simulink model "plantaNeural"  (Simulink 7.4)
settings: Solver=ode45  StartTime=0.0  StopTime=10000  RelTol=1e-3
undefined symbols (not defined in the file or in its folder): now
libraries: neural x29, simulink_extras x2
settings Model: Creator=marco  LastModifiedBy=marco

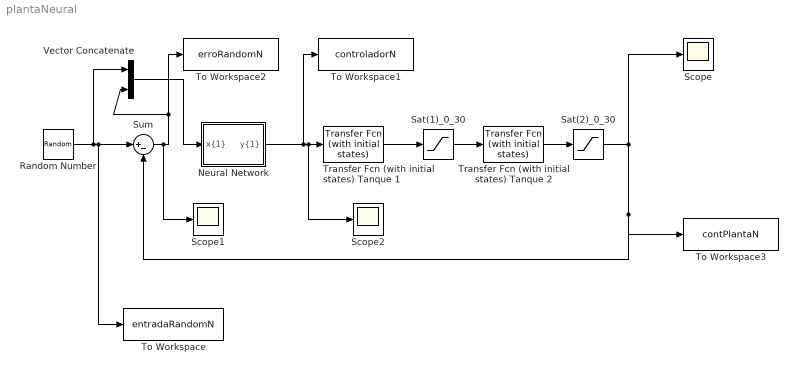
== system plantaNeural ==
  Neural Network : Subsystem
  Random Number : RandomNumber  Mean=15  Variance=15  Seed=round(now)  SampleTime=500
  Sat(1)_0_30 : Saturate  UpperLimit=30  LowerLimit=0  SampleTime=0.1  OutDataType=fixdt(1, 16)  OutScaling=2^0
  Sat(2)_0_30 : Saturate  UpperLimit=30  LowerLimit=0  SampleTime=0.1  OutDataType=fixdt(1, 16)  OutScaling=2^0
  Scope : Scope
  Scope1 : Scope
  Scope2 : Scope
      settings: YMin=4  YMax=5.5  SaveName=ScopeData2
  Sum : Sum  Inputs=|+-  OutDataType=fixdt(1, 16)  OutScaling=2^0  SampleTime=0.1
  To Workspace : ToWorkspace  VariableName=entradaRandomN  SampleTime=0.1  SaveFormat=Array
  To Workspace1 : ToWorkspace  VariableName=controladorN  SampleTime=0.1  SaveFormat=Array
  To Workspace2 : ToWorkspace  VariableName=erroRandomN  SampleTime=0.1  SaveFormat=Array
  To Workspace3 : ToWorkspace  VariableName=contPlantaN  SampleTime=0.1  SaveFormat=Array
  Transfer Fcn (with initial states) Tanque 1 : simulink_extras/Additional Linear/Transfer Fcn (with initial states)  SystemSampleTime=-1  N=[0.2964]  D="[1  0.0656]"  X0=0
  Transfer Fcn (with initial states) Tanque 2 : simulink_extras/Additional Linear/Transfer Fcn (with initial states)  SystemSampleTime=-1  N=[0.0656]  D="[1  0.0656]"  X0=0
  Vector Concatenate : Concatenate  Mode=Vector
  wires:
  Transfer Fcn (with initial states) Tanque 1/1 -> Sat(1)_0_30/1
  Sum/1 -> Scope1/1, To Workspace2/1, Vector Concatenate/2
  Transfer Fcn (with initial states) Tanque 2/1 -> Sat(2)_0_30/1
  Neural Network/1("y{1}") -> To Workspace1/1, Transfer Fcn (with initial states) Tanque 1/1, Scope2/1
  Random Number/1 -> To Workspace/1, Sum/1, Vector Concatenate/1
  Sat(1)_0_30/1 -> Transfer Fcn (with initial states) Tanque 2/1
  Sat(2)_0_30/1 -> Scope/1, Sum/2, To Workspace3/1
  Vector Concatenate/1 -> Neural Network/1("x{1}")

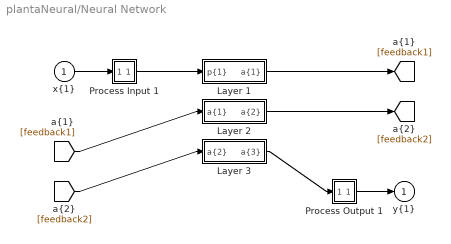
== system plantaNeural/Neural Network ==
  "x{1}" : Inport  PortDimensions=2  SampleTime=1
  Layer 1 : Subsystem
  Layer 2 : Subsystem
  Layer 3 : Subsystem
  Process Input 1 : Subsystem
  Process Output 1 : Subsystem
  "y{1}" : Outport  InitialOutput=0
  wires:
  "x{1}"/1 -> Process Input 1/1(x)
  Process Output 1/1(y) -> "y{1}"/1
  Process Input 1/1(p) -> Layer 1/1("p{1}")
  Layer 1/1("a{1}") -> [feedback1]
  [feedback1] -> Layer 2/1("a{1} ")
  Layer 2/1("a{2}") -> [feedback2]
  [feedback2] -> Layer 3/1("a{2} ")
  Layer 3/1("a{3}") -> Process Output 1/1(a)

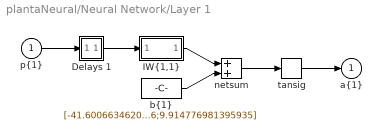
== system plantaNeural/Neural Network/Layer 1 ==
  "p{1}" : Inport  PortDimensions=2  SampleTime=1
  Delays 1 : Subsystem
      mask Display: disp('TDL')
  "IW{1,1}" : Subsystem
      mask Display: disp('weight')
  "b{1}" : Constant  Value=[-41.600663462015341;-13.867070844846031;-1.0368982298681877;-25.663752606811631;65.028796099680704;3.5608850337005888;6.4712500253222389;61.743011559162341;7.1136119483346736;9.914776981395935]
      mask Display: disp('bias')
  netsum : Sum  Inputs=2  OutDataType=sfix(16)  OutScaling=2^0  SaturateOnIntegerOverflow=on  InputSameDT=on  OutDataTypeStr=Inherit: Same as first input
  tansig : neural/Transfer Functions/tansig  SystemSampleTime=-1
  "a{1}" : Outport  InitialOutput=[0;0;0;0;0;0;0;0;0;0]
  wires:
  "p{1}"/1 -> Delays 1/1("p{1}")
  Delays 1/1("pd{1,1}") -> "IW{1,1}"/1("pd{1,1}")
  "IW{1,1}"/1("iz{1,1}") -> netsum/1
  "b{1}"/1 -> netsum/2
  netsum/1 -> tansig/1
  tansig/1 -> "a{1}"/1

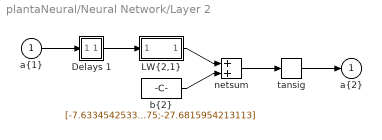
== system plantaNeural/Neural Network/Layer 2 ==
  "a{1} " : Inport  PortDimensions=10  SampleTime=1
  Delays 1 : Subsystem
      mask Display: disp('TDL')
  "LW{2,1}" : Subsystem
      mask Display: disp('weight')
  "b{2}" : Constant  Value=[-7.6334542533188312;-15.605769004106929;9.5386103916769969;-0.097339973816270103;36.782799143926788;8.2018066341292926;15.153030458866333;4.2679298498601739;36.406304506237475;-27.6815954213113]
      mask Display: disp('bias')
  netsum : Sum  Inputs=2  OutDataType=sfix(16)  OutScaling=2^0  SaturateOnIntegerOverflow=on  InputSameDT=on  OutDataTypeStr=Inherit: Same as first input
  tansig : neural/Transfer Functions/tansig  SystemSampleTime=-1
  "a{2}" : Outport  InitialOutput=[0;0;0;0;0;0;0;0;0;0]
  wires:
  "a{1} "/1 -> Delays 1/1("p{2}")
  Delays 1/1("pd{2,1}") -> "LW{2,1}"/1("ad{2,1}")
  "LW{2,1}"/1("lz{2,1}") -> netsum/1
  "b{2}"/1 -> netsum/2
  netsum/1 -> tansig/1
  tansig/1 -> "a{2}"/1

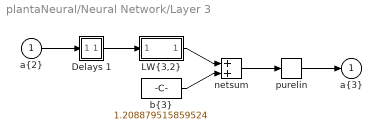
== system plantaNeural/Neural Network/Layer 3 ==
  "a{2} " : Inport  PortDimensions=10  SampleTime=1
  Delays 1 : Subsystem
      mask Display: disp('TDL')
  "LW{3,2}" : Subsystem
      mask Display: disp('weight')
  "b{3}" : Constant  Value=1.208879515859524
      mask Display: disp('bias')
  netsum : Sum  Inputs=2  OutDataType=sfix(16)  OutScaling=2^0  SaturateOnIntegerOverflow=on  InputSameDT=on  OutDataTypeStr=Inherit: Same as first input
  purelin : neural/Transfer Functions/purelin  SystemSampleTime=-1
  "a{3}" : Outport  InitialOutput=0
  wires:
  "a{2} "/1 -> Delays 1/1("p{3}")
  Delays 1/1("pd{3,2}") -> "LW{3,2}"/1("ad{3,2}")
  "LW{3,2}"/1("lz{3,2}") -> netsum/1
  "b{3}"/1 -> netsum/2
  netsum/1 -> purelin/1
  purelin/1 -> "a{3}"/1

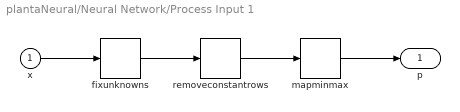
== system plantaNeural/Neural Network/Process Input 1 ==
  x : Inport  PortDimensions=2  SampleTime=1
  fixunknowns : neural/Processing Functions/fixunknowns  SystemSampleTime=-1  dummy=0
  mapminmax : neural/Processing Functions/mapminmax  SystemSampleTime=-1  xmin=[22.37203801183;-6.51958225632998]  xmax=[29.5106040109867;23.0027682108523]  ymin=-1  ymax=1
  removeconstantrows : neural/Processing Functions/removeconstantrows  SystemSampleTime=-1  inputSize=2  keep=[1 2]
  p : Outport  PortDimensions=2  SampleTime=1
  wires:
  x/1 -> fixunknowns/1
  fixunknowns/1 -> removeconstantrows/1
  removeconstantrows/1 -> mapminmax/1
  mapminmax/1 -> p/1

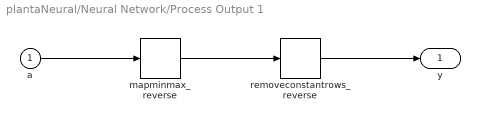
== system plantaNeural/Neural Network/Process Output 1 ==
  a : Inport  PortDimensions=1  SampleTime=1
  mapminmax_reverse : neural/Processing Functions/mapminmax_reverse  SystemSampleTime=-1  xmin=-15  xmax=15  ymin=-1  ymax=1
  removeconstantrows_reverse : neural/Processing Functions/removeconstantrows_reverse  SystemSampleTime=-1  inputSize=1  constants=zeros(0,1)  rearrange=1
  y : Outport  PortDimensions=1  SampleTime=1
  wires:
  a/1 -> mapminmax_reverse/1
  mapminmax_reverse/1 -> removeconstantrows_reverse/1
  removeconstantrows_reverse/1 -> y/1

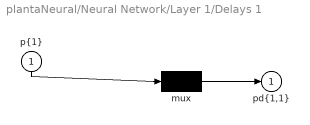
== system plantaNeural/Neural Network/Layer 1/Delays 1 ==
  "p{1}" : Inport  PortDimensions=2  SampleTime=1
  mux : Mux  Inputs=1
  "pd{1,1}" : Outport
  wires:
  "p{1}"/1 -> mux/1
  mux/1 -> "pd{1,1}"/1

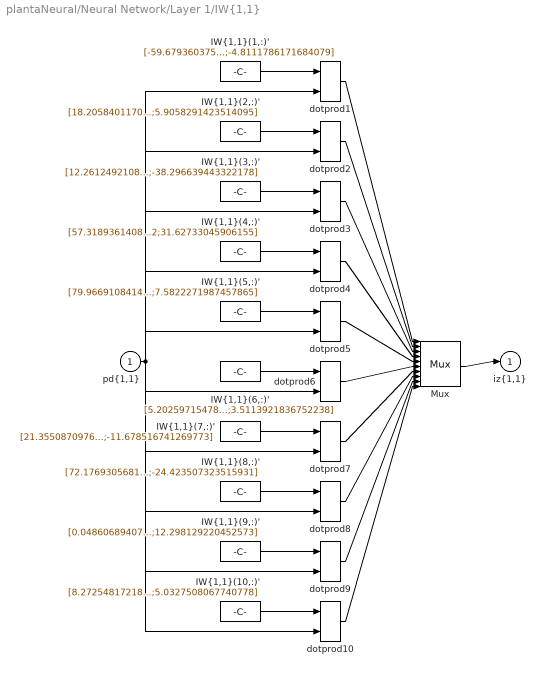
== system plantaNeural/Neural Network/Layer 1/IW{1,1} ==
  "pd{1,1}" : Inport  PortDimensions=2  SampleTime=1
  "IW{1,1}(1,:)'" : Constant  Value=[-59.679360375161757;-4.8111786171684079]
      mask Display: disp('weights')
  "IW{1,1}(10,:)'" : Constant  Value=[8.2725481721899286;5.0327508067740778]
      mask Display: disp('weights')
  "IW{1,1}(2,:)'" : Constant  Value=[18.205840117067901;5.9058291423514095]
      mask Display: disp('weights')
  "IW{1,1}(3,:)'" : Constant  Value=[12.26124921081548;-38.296639443322178]
      mask Display: disp('weights')
  "IW{1,1}(4,:)'" : Constant  Value=[57.318936140845892;31.62733045906155]
      mask Display: disp('weights')
  "IW{1,1}(5,:)'" : Constant  Value=[79.966910841416151;7.5822271987457865]
      mask Display: disp('weights')
  "IW{1,1}(6,:)'" : Constant  Value=[5.2025971547884202;3.5113921836752238]
      mask Display: disp('weights')
  "IW{1,1}(7,:)'" : Constant  Value=[21.355087097600556;-11.678516741269773]
      mask Display: disp('weights')
  "IW{1,1}(8,:)'" : Constant  Value=[72.17693056814872;-24.423507323515931]
      mask Display: disp('weights')
  "IW{1,1}(9,:)'" : Constant  Value=[0.048606894072706332;12.298129220452573]
      mask Display: disp('weights')
  Mux : Mux  Inputs=10
  dotprod{1..10} (10 alike) : neural/Weight Functions/dotprod  SystemSampleTime=-1
  "iz{1,1}" : Outport
  wires:
  "IW{1,1}(1,:)'"/1 -> dotprod1/1
  "pd{1,1}"/1 -> dotprod1/2, dotprod2/2, dotprod3/2, dotprod4/2, dotprod5/2, dotprod6/2, dotprod7/2, dotprod8/2, dotprod9/2, dotprod10/2
  dotprod1/1 -> Mux/1
  "IW{1,1}(2,:)'"/1 -> dotprod2/1
  dotprod2/1 -> Mux/2
  "IW{1,1}(3,:)'"/1 -> dotprod3/1
  dotprod3/1 -> Mux/3
  "IW{1,1}(4,:)'"/1 -> dotprod4/1
  dotprod4/1 -> Mux/4
  "IW{1,1}(5,:)'"/1 -> dotprod5/1
  dotprod5/1 -> Mux/5
  "IW{1,1}(6,:)'"/1 -> dotprod6/1
  dotprod6/1 -> Mux/6
  "IW{1,1}(7,:)'"/1 -> dotprod7/1
  dotprod7/1 -> Mux/7
  "IW{1,1}(8,:)'"/1 -> dotprod8/1
  dotprod8/1 -> Mux/8
  "IW{1,1}(9,:)'"/1 -> dotprod9/1
  dotprod9/1 -> Mux/9
  "IW{1,1}(10,:)'"/1 -> dotprod10/1
  dotprod10/1 -> Mux/10
  Mux/1 -> "iz{1,1}"/1

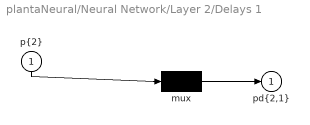
== system plantaNeural/Neural Network/Layer 2/Delays 1 ==
  "p{2}" : Inport  PortDimensions=10  SampleTime=1
  mux : Mux  Inputs=1
  "pd{2,1}" : Outport
  wires:
  "p{2}"/1 -> mux/1
  mux/1 -> "pd{2,1}"/1

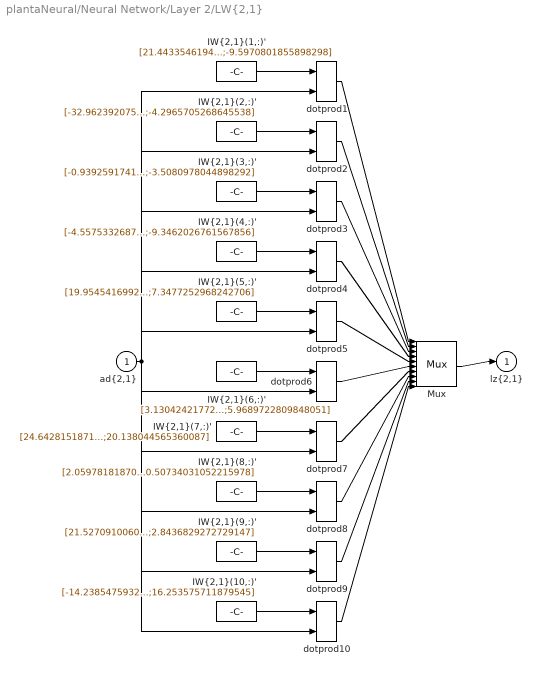
== system plantaNeural/Neural Network/Layer 2/LW{2,1} ==
  "ad{2,1}" : Inport  PortDimensions=10  SampleTime=1
  "IW{2,1}(1,:)'" : Constant  Value=[21.443354619468462;-1.3006422170219611;7.8955057727334754;-4.7979796157139463;-25.898773850093161;-3.1265477241198587;-33.886964502007594;7.8665509727248129;5.0238934577656122;-9.5970801855898298]
      mask Display: disp('weights')
  "IW{2,1}(10,:)'" : Constant  Value=[-14.238547593274664;42.105928129329328;-77.196582677683395;-27.448455327920765;38.673784847710017;75.547984645249272;66.867314859757926;26.392337906608308;-6.9796643502251374;16.253575711879545]
      mask Display: disp('weights')
  "IW{2,1}(2,:)'" : Constant  Value=[-32.962392075897931;-20.153864455929828;-9.7633107877471623;39.465729228039216;-9.5385756012289811;-72.215836359371636;5.1870396695462837;17.760679452039696;-62.831055912876309;-4.2965705268645538]
      mask Display: disp('weights')
  "IW{2,1}(3,:)'" : Constant  Value=[-0.93925917415433302;-2.1121683627624659;18.321533288736973;-2.1121350388538596;-32.64063375843083;-0.082227510725482206;-0.053308046914458243;2.1867023554264611;-1.8934095863755567;-3.5080978044898292]
      mask Display: disp('weights')
  "IW{2,1}(4,:)'" : Constant  Value=[-4.5575332687997614;6.564948030885378;6.2249388677457649;-12.19791938596962;8.7687324360660952;13.298488776720923;1.1606561206397161;7.0780288866158694;-1.7261832076371659;-9.3462026761567856]
      mask Display: disp('weights')
  "IW{2,1}(5,:)'" : Constant  Value=[19.954541699244142;-82.519813861266172;7.5863885346027748;17.78262506166444;35.871696191680805;-4.3259342125193072;7.9743771576504381;-19.930082687281338;5.6241815886969349;7.3477252968242706]
      mask Display: disp('weights')
  "IW{2,1}(6,:)'" : Constant  Value=[3.1304242177289074;-34.579832915356235;2.9437994208273297;8.865101748692048;5.2342992632779382;-11.465825065558862;2.4837998140417357;-2.2714157367541423;-3.2081770594202146;5.9689722809848051]
      mask Display: disp('weights')
  "IW{2,1}(7,:)'" : Constant  Value=[24.642815187128299;-21.698895502716027;-5.2629617573667575;17.413853751335953;-33.363267640689564;104.84978734729668;-18.080830187475989;-19.048008231174531;50.250486908270815;20.138044565360087]
      mask Display: disp('weights')
  "IW{2,1}(8,:)'" : Constant  Value=[2.0597818187068966;-0.31382842787036613;-0.0050154807493239589;0.13974099503462253;0.99054211211615395;-0.18124225565312488;0.41232083732936464;-1.8036724102957487;-5.0426437994966982;0.50734031052215978]
      mask Display: disp('weights')
  "IW{2,1}(9,:)'" : Constant  Value=[21.527091006027007;-7.8145360671285333;4.9067209119409743;15.62613610401363;136.61659342280001;-20.511573746758557;-11.485462041142192;-49.047173900407266;-2.3604346155640461;2.8436829272729147]
      mask Display: disp('weights')
  Mux : Mux  Inputs=10
  dotprod{1..10} (10 alike) : neural/Weight Functions/dotprod  SystemSampleTime=-1
  "lz{2,1}" : Outport
  wires:
  "IW{2,1}(1,:)'"/1 -> dotprod1/1
  "ad{2,1}"/1 -> dotprod1/2, dotprod2/2, dotprod3/2, dotprod4/2, dotprod5/2, dotprod6/2, dotprod7/2, dotprod8/2, dotprod9/2, dotprod10/2
  dotprod1/1 -> Mux/1
  "IW{2,1}(2,:)'"/1 -> dotprod2/1
  dotprod2/1 -> Mux/2
  "IW{2,1}(3,:)'"/1 -> dotprod3/1
  dotprod3/1 -> Mux/3
  "IW{2,1}(4,:)'"/1 -> dotprod4/1
  dotprod4/1 -> Mux/4
  "IW{2,1}(5,:)'"/1 -> dotprod5/1
  dotprod5/1 -> Mux/5
  "IW{2,1}(6,:)'"/1 -> dotprod6/1
  dotprod6/1 -> Mux/6
  "IW{2,1}(7,:)'"/1 -> dotprod7/1
  dotprod7/1 -> Mux/7
  "IW{2,1}(8,:)'"/1 -> dotprod8/1
  dotprod8/1 -> Mux/8
  "IW{2,1}(9,:)'"/1 -> dotprod9/1
  dotprod9/1 -> Mux/9
  "IW{2,1}(10,:)'"/1 -> dotprod10/1
  dotprod10/1 -> Mux/10
  Mux/1 -> "lz{2,1}"/1

== system plantaNeural/Neural Network/Layer 3/Delays 1 ==
  "p{3}" : Inport  PortDimensions=10  SampleTime=1
  mux : Mux  Inputs=1
  "pd{3,2}" : Outport
  wires:
  "p{3}"/1 -> mux/1
  mux/1 -> "pd{3,2}"/1

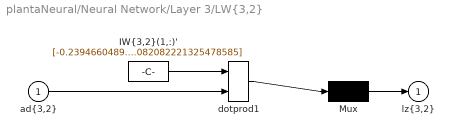
== system plantaNeural/Neural Network/Layer 3/LW{3,2} ==
  "ad{3,2}" : Inport  PortDimensions=10  SampleTime=1
  "IW{3,2}(1,:)'" : Constant  Value=[-0.23946604895932105;-0.083078428122546871;-0.75357468216088375;-0.54738167813523653;-0.57905518422487101;0.052222389670158818;-0.015918502219387554;-0.3028157350192523;-0.41383242519324592;-0.082082221325478585]
      mask Display: disp('weights')
  Mux : Mux  Inputs=1
  dotprod1 : neural/Weight Functions/dotprod  SystemSampleTime=-1
  "lz{3,2}" : Outport
  wires:
  "IW{3,2}(1,:)'"/1 -> dotprod1/1
  "ad{3,2}"/1 -> dotprod1/2
  dotprod1/1 -> Mux/1
  Mux/1 -> "lz{3,2}"/1
